simulink model "launchControl"  (R2024b)
settings: Solver=VariableStepAuto  StartTime=0.0  StopTime=10.0  RelTol=1e-3
values from neighbouring files (symbols this model uses):
  g = 9.81    [constants.mat]    (also in vehcileConstants2025.m)
  lr = 0.859026    [constants.mat]    (also in vehcileConstants2025.m)
  m =     [constants.mat]
  torque_vs_RPM_breakpoints = [0 5500 6048 6500]    [constants.mat]    (also in vehcileConstants2025.m = [0, 5500, 6048, 6500])
  torque_vs_RPM_table = [220 220 170 0]    [constants.mat]    (also in vehcileConstants2025.m = [220, 220, 170, 0])
  wheel =     [constants.mat]
libraries: simulink x1, autolibshared x1
settings Model: Creator=nhola  LastModifiedBy=nhola
settings DataIOCC: ExternalInput=[Tire, Parameter]
settings DebuggingCC: UnderSpecifiedDimensionMsg=warning

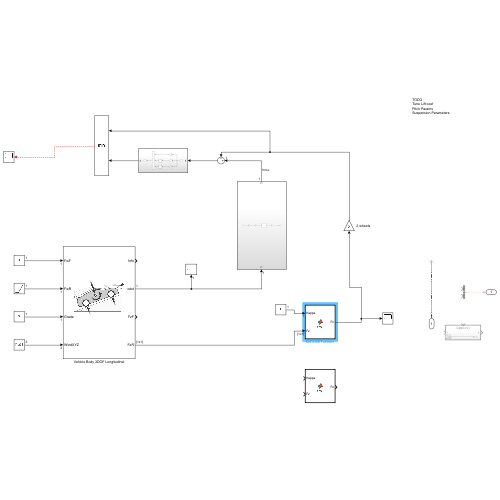
[thumbnail: Simulink's stored preview of the top-level diagram]
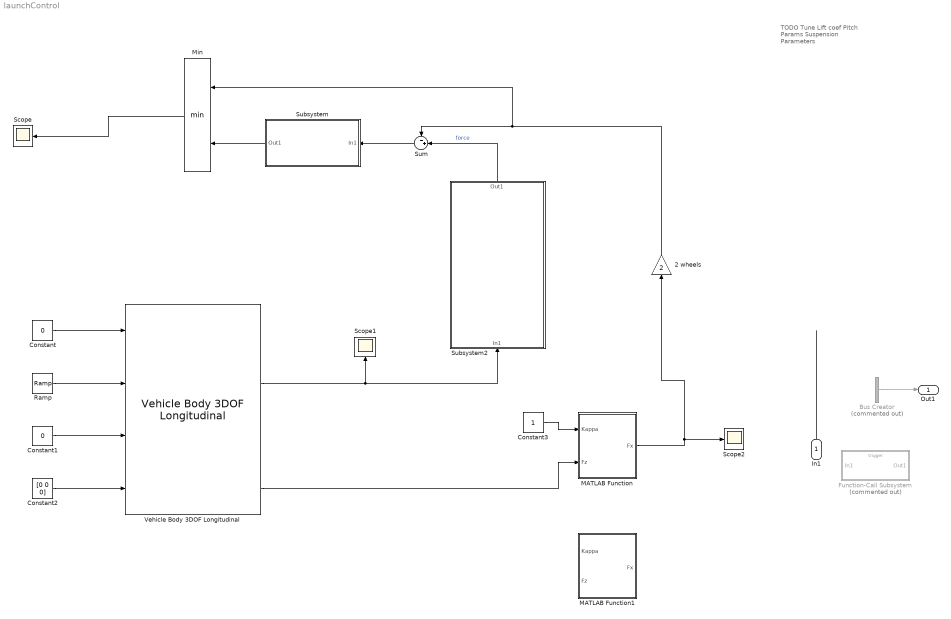
== system launchControl ==
  note: TODO
      | Tune Lift coef
      | Pitch Params
      | Suspension Parameters
  In1 : Inport
  2 wheels : Gain  Gain=2
  Bus Creator : BusCreator  Commented=on  Inputs=2
  Constant : Constant  Value=0
  Constant1 : Constant  Value=0
  Constant2 : Constant  Value=[0 0 0]
  Constant3 : Constant
  Function-Call Subsystem : Subsystem  Commented=on  TreatAsAtomicUnit=on
  MATLAB Function : MATLAB Function  TreatAsAtomicUnit=on
  MATLAB Function1 : MATLAB Function  TreatAsAtomicUnit=on
  Min : MinMax  Inputs=2
  Ramp : simulink/Sources/Ramp  slope=1  start=0  InitialOutput=0
  Scope : Scope
  Scope1 : Scope
  Scope2 : Scope
  Subsystem : Subsystem
  Subsystem2 : Subsystem
  Sum : Sum  Inputs=-+|
  Vehicle Body 3DOF Longitudinal : autolibshared/Vehicle Body 3DOF Longitudinal  VariantControl=SL  groundType=Grade angle  aMode=2  extFMode=off  extMMode=off  extTamb=off  NF=2  NR=2  m=m.total  a=lf  b=lr  h=hCG  Cd=Cd  Af=A_ref  x_o=0  xdot_o=0  Cl=.1  z_o=-.35  zdot_o=0  Iyy=3500  Cpm=.1  theta_o=0  q_o=0  FskF=[-50, -1, 0, 2, 3, 52].*1.5e4  dzsF=[-5e-3, -1e-4, 0, .2, .2001, .2051]  FsbF=[-10000 -100 -10 0 10 100 10000]  dzdotsF=[-10 -1 -.1 0 .1 1 10]  FskR=[-50, -1, 0, 2, 3, 52].*1e4  dzsR=[-5e-3, -1e-4, 0, .2, .2001, .2051]  FsbR=[-10000 -100 -10 0 10 100 10000]  dzdotsR=[-10 -1 -.1 0 .1 1 10]  Pabs=101325  T=273  g=g  blkID=0
      settings: LibrarySourceBlock=vehdynlibeom/Vehicle Body 3DOF Longitudinal
  Out1 : Outport
  wires:
  Constant/1 -> Vehicle Body 3DOF Longitudinal/1
  Constant2/1 -> Vehicle Body 3DOF Longitudinal/4
  Constant1/1 -> Vehicle Body 3DOF Longitudinal/3
  Vehicle Body 3DOF Longitudinal/2 -> Scope1/1, Subsystem2/1(In1)
  Vehicle Body 3DOF Longitudinal/4 -> MATLAB Function/2(Fz)
  Subsystem/1(Out1) -> Min/2
  Subsystem2/1(Out1) -> Sum/2  "force"
  Min/1 -> Scope/1
  2 wheels/1 -> Min/1, Sum/1
  Ramp/1 -> Vehicle Body 3DOF Longitudinal/2
  Sum/1 -> Subsystem/1(In1)
  Bus Creator/1 -> Out1/1
  In1/1 -> ?
  MATLAB Function/1(Fx) -> 2 wheels/1, Scope2/1
  Constant3/1 -> MATLAB Function/1(Kappa)

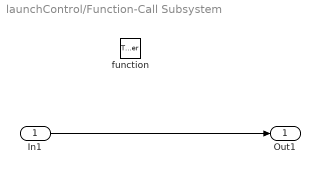
== system launchControl/Function-Call Subsystem ==
  In1 : Inport
  function : TriggerPort  TriggerType=function-call  VariantControl=(inherit)
  Out1 : Outport
  wires:
  In1/1 -> Out1/1

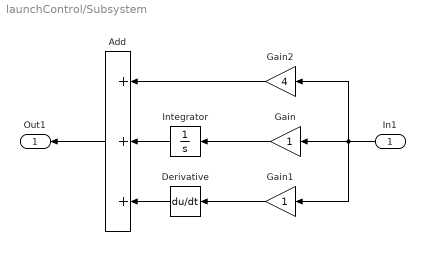
== system launchControl/Subsystem ==
  In1 : Inport
  Add : Sum  Inputs=+++
  Derivative : Derivative
  Gain : Gain
  Gain1 : Gain
  Gain2 : Gain  Gain=4
  Integrator : Integrator
  Out1 : Outport
  wires:
  Gain/1 -> Integrator/1
  Integrator/1 -> Add/2
  Gain2/1 -> Add/1
  Derivative/1 -> Add/3
  Gain1/1 -> Derivative/1
  In1/1 -> Gain/1, Gain1/1, Gain2/1
  Add/1 -> Out1/1

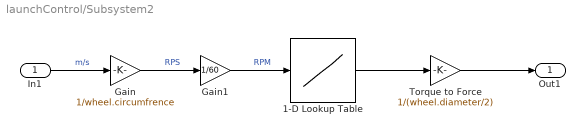
== system launchControl/Subsystem2 ==
  In1 : Inport
  1-D Lookup Table : Lookup_n-D  NumberOfTableDimensions=1  BreakpointsForDimension1=torque_vs_RPM_breakpoints  Table=torque_vs_RPM_table  InternalRulePriority=Speed  RndMeth=Simplest
  Gain : Gain  Gain=1/wheel.circumfrence
  Gain1 : Gain  Gain=1/60
  Torque to Force : Gain  Gain=1/(wheel.diameter/2)
  Out1 : Outport
  wires:
  In1/1 -> Gain/1  "m/s"
  Gain/1 -> Gain1/1  "RPS"
  Gain1/1 -> 1-D Lookup Table/1  "RPM"
  1-D Lookup Table/1 -> Torque to Force/1
  Torque to Force/1 -> Out1/1

== matlab function launchControl/MATLAB Function1 ==
  data: Kappa input; Fx output; Fz input
function Fx = fcn(Kappa, Fz)
Pi = 70;
Inc = 0;

dFz = (Fz - Parameter.Pacejka.Fzo) ./ Parameter.Pacejka.Fzo;
dPi = (Pi - Parameter.Pacejka.Pio) ./ Parameter.Pacejka.Pio;

Cx = Parameter.Pacejka.p.C.x(1) .* Parameter.Pacejka.L.C.x;

Dx = (Parameter.Pacejka.p.D.x(1) + Parameter.Pacejka.p.D.x(2).*dFz) .* ...
     (1 + Parameter.Pacejka.p.P.x(3).*dPi + Parameter.Pacejka.p.P.x(4).*dPi.^2) .* ...
     (1 - Parameter.Pacejka.p.D.x(3).*Inc.^2).*Fz .* Parameter.Pacejka.L.mu.x;

Ex = ( Parameter.Pacejka.p.E.x(1) + Parameter.Pacejka.p.E.x(2).*dFz ...
    + Parameter.Pacejka.p.E.x(3).*dFz.^2 ) .* ( 1 - Parameter.Pacejka.p.E.x(4).*sign(Kappa) ) .* ...
    Parameter.Pacejka.L.E.x;

Kxk = Fz.*(Parameter.Pacejka.p.K.x(1) + Parameter.Pacejka.p.K.x(2).*dFz ) .* ...
    exp( Parameter.Pacejka.p.K.x(3) .* dFz ) .* ...
    (1 + Parameter.Pacejka.p.P.x(1).*dPi + Parameter.Pacejka.p.P.x(2).*dPi.^2) .* ...
    Parameter.Pacejka.L.K.x.k;

Bx = Kxk ./ ( Cx.*Dx );

Vx = Fz.*(Parameter.Pacejka.p.V.x(1) + Parameter.Pacejka.p.V.x(2).*dFz ) .* ...
    Parameter.Pacejka.L.V.x;

Hx = (Parameter.Pacejka.p.H.x(1) + Parameter.Pacejka.p.H.x(2).*dFz) .* ...
    Parameter.Pacejka.L.H.x;

Fx = Dx .* sin( Cx .* atan( (1-Ex) .* Bx.*(Kappa + Hx) + ...
    Ex.*atan( Bx.*(Kappa + Hx) ) ) ) + Vx;



end

== matlab function launchControl/MATLAB Function ==
  data: Kappa input; Fx output; Fz input; Parameter parameter
function Fx = fcn(Kappa, Fz, Parameter)
Pi = 70;
Inc = 0;

dFz = (Fz - Parameter.Pacejka.Fzo) ./ Parameter.Pacejka.Fzo;
dPi = (Pi - Parameter.Pacejka.Pio) ./ Parameter.Pacejka.Pio;

Cx = Parameter.Pacejka.p.C.x(1) .* Parameter.Pacejka.L.C.x;

Dx = (Parameter.Pacejka.p.D.x(1) + Parameter.Pacejka.p.D.x(2).*dFz) .* ...
     (1 + Parameter.Pacejka.p.P.x(3).*dPi + Parameter.Pacejka.p.P.x(4).*dPi.^2) .* ...
     (1 - Parameter.Pacejka.p.D.x(3).*Inc.^2).*Fz .* Parameter.Pacejka.L.mu.x;

Ex = ( Parameter.Pacejka.p.E.x(1) + Parameter.Pacejka.p.E.x(2).*dFz ...
    + Parameter.Pacejka.p.E.x(3).*dFz.^2 ) .* ( 1 - Parameter.Pacejka.p.E.x(4).*sign(Kappa) ) .* ...
    Parameter.Pacejka.L.E.x;

Kxk = Fz.*(Parameter.Pacejka.p.K.x(1) + Parameter.Pacejka.p.K.x(2).*dFz ) .* ...
    exp( Parameter.Pacejka.p.K.x(3) .* dFz ) .* ...
    (1 + Parameter.Pacejka.p.P.x(1).*dPi + Parameter.Pacejka.p.P.x(2).*dPi.^2) .* ...
    Parameter.Pacejka.L.K.x.k;

Bx = Kxk ./ ( Cx.*Dx );

Vx = Fz.*(Parameter.Pacejka.p.V.x(1) + Parameter.Pacejka.p.V.x(2).*dFz ) .* ...
    Parameter.Pacejka.L.V.x;

Hx = (Parameter.Pacejka.p.H.x(1) + Parameter.Pacejka.p.H.x(2).*dFz) .* ...
    Parameter.Pacejka.L.H.x;

Fx = Dx .* sin( Cx .* atan( (1-Ex) .* Bx.*(Kappa + Hx) + ...
    Ex.*atan( Bx.*(Kappa + Hx) ) ) ) + Vx;



end
